simulink model "DiffEstimator"  (R2017a)
settings: Solver=VariableStepAuto  StartTime=0.0  StopTime=3  RelTol=1e-3
values from neighbouring files (symbols this model uses):
  h_A = 360/(N*z)    (= 1.53649167734)    [diffEstimator.m]
  h_T = 1/(N*n*z/60)    (= 0.00426803243705)    [diffEstimator.m]
  n = 60    [diffEstimator.m]
libraries: simulink x2
settings Model: Creator=Vsevolod  LastModifiedBy=Vsevolod

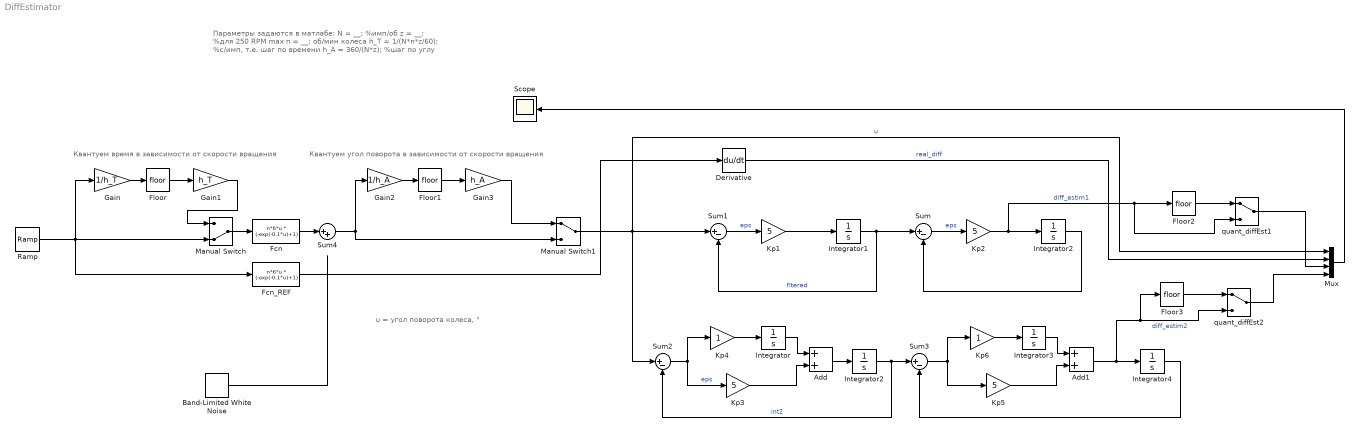
== system DiffEstimator ==
  note: u = угол поворота колеса, °
  note: Параметры задаются в матлабе:
      |
      | N = __; %имп/об
      | z = __; %для 250 RPM max
      | n = __; об/мин колеса
      | h_T = 1/(N*n*z/60); %с/имп, т.е. шаг по времени
      | h_A = 360/(N*z); %шаг по углу
  note: Квантуем угол поворота в зависимости от скорости вращения
  note: Квантуем время в зависимости от скорости вращения
  Add : Sum
  Add1 : Sum
  Band-Limited White Noise : simulink/Sources/Band-Limited White Noise  Cov=[0.001]  Ts=0.001  seed=[23341]
  Derivative : Derivative
  Fcn : Fcn  Expr=n*6*u * (-exp(-0.1*u)+1)
  Fcn_REF : Fcn  Expr=n*6*u * (-exp(-0.1*u)+1)
  Floor{,1..3} (4 alike) : Rounding
  Gain : Gain  Gain=1/h_T
  Gain1 : Gain  Gain=h_T
  Gain2 : Gain  Gain=1/h_A
  Gain3 : Gain  Gain=h_A
  Integrator{,1..4} (5 alike) : Integrator
  "Integrator2 " : Integrator
  Kp{1..3,5} (4 alike) : Gain  Gain=5
  Kp4 : Gain
  Kp6 : Gain
  Manual Switch : ManualSwitch  CurrentSetting=0
  Manual Switch1 : ManualSwitch
  Mux : Mux
  Ramp : simulink/Sources/Ramp  slope=1  start=0  X0=0
  Scope : Scope
  Sum{,1..3} (4 alike) : Sum  Inputs=|+-
  Sum4 : Sum  Inputs=|++
  quant_diffEst1 : ManualSwitch
  quant_diffEst2 : ManualSwitch
  wires:
  Manual Switch1/1 -> Sum2/1, Mux/1, Sum1/1  "u"
  Sum/1 -> Kp2/1  "eps"
  Kp2/1 -> quant_diffEst1/2, Floor2/1, "Integrator2 "/1  "diff_estim1"
  "Integrator2 "/1 -> Sum/2
  Mux/1 -> Scope/1
  Integrator1/1 -> Sum/1, Sum1/2  "fltered"
  Derivative/1 -> Mux/2  "real_diff"
  Kp1/1 -> Integrator1/1
  Sum1/1 -> Kp1/1  "eps"
  Sum2/1 -> Kp4/1, Kp3/1  "eps"
  Kp4/1 -> Integrator/1
  Integrator/1 -> Add/1
  Kp3/1 -> Add/2
  Add/1 -> Integrator2/1
  Integrator2/1 -> Sum3/1, Sum2/2  "int2"
  Integrator3/1 -> Add1/1
  Kp6/1 -> Integrator3/1
  Kp5/1 -> Add1/2
  Add1/1 -> quant_diffEst2/2, Floor3/1, Integrator4/1  "diff_estim2"
  Integrator4/1 -> Sum3/2
  Sum3/1 -> Kp6/1, Kp5/1
  Band-Limited White Noise/1 -> ?
  Ramp/1 -> Fcn_REF/1, Manual Switch/2, Gain/1
  Gain/1 -> Floor/1
  Manual Switch/1 -> Fcn/1
  Floor/1 -> Gain1/1
  Gain1/1 -> Manual Switch/1
  Fcn_REF/1 -> Derivative/1
  Sum4/1 -> Gain2/1, Manual Switch1/2
  Gain2/1 -> Floor1/1
  Floor1/1 -> Gain3/1
  Gain3/1 -> Manual Switch1/1
  Fcn/1 -> Sum4/1
  Floor2/1 -> quant_diffEst1/1
  Floor3/1 -> quant_diffEst2/1
  quant_diffEst1/1 -> Mux/3
  quant_diffEst2/1 -> Mux/4
